simulink model "nonlinear_pid"  (R2021b)
settings: Solver=VariableStepAuto  StartTime=0.0  StopTime=60  RelTol=1e-3
libraries: slpidlib x6
settings Model: Creator=QP  LastModifiedBy=QP

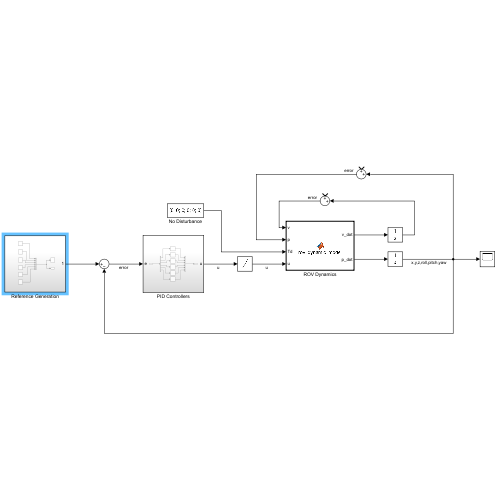
[thumbnail: Simulink's stored preview of the top-level diagram]
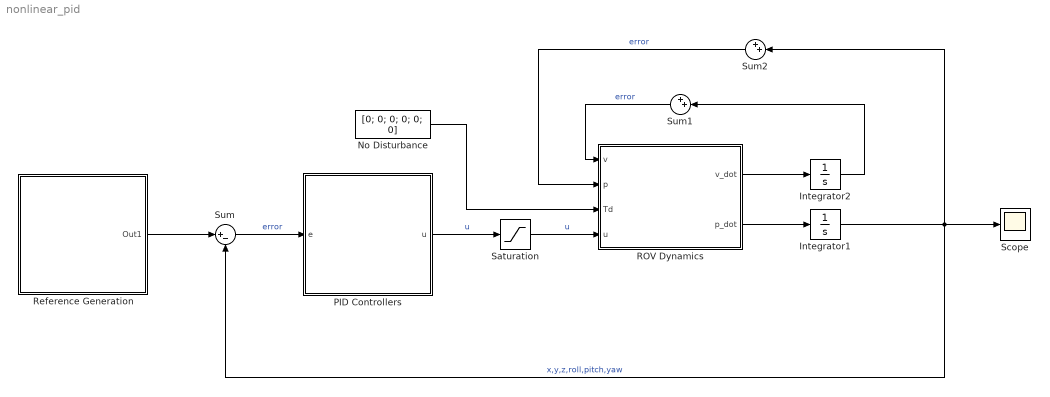
== system nonlinear_pid ==
  Integrator1 : Integrator
  Integrator2 : Integrator
  No Disturbance : Constant  Value=[0; 0; 0; 0; 0; 0]
  PID Controllers : Subsystem
  ROV Dynamics : MATLAB Function  TreatAsAtomicUnit=on
  Reference Generation : Subsystem
  Saturation : Saturate  UpperLimit=1  LowerLimit=-1
  Scope : Scope
  Sum : Sum  Inputs=|+-
  Sum1 : Sum  Inputs=++|
  Sum2 : Sum  Inputs=++|
  wires:
  PID Controllers/1(u) -> Saturation/1  "u"
  Reference Generation/1(Out1) -> Sum/1
  Sum/1 -> PID Controllers/1(e)  "error"
  Saturation/1 -> ROV Dynamics/4(u)  "u"
  No Disturbance/1 -> ROV Dynamics/3(Td)
  ROV Dynamics/2(p_dot) -> Integrator1/1
  ROV Dynamics/1(v_dot) -> Integrator2/1
  Integrator1/1 -> Sum2/2, Scope/1, Sum/2  "x,y,z,roll,pitch,yaw"
  Integrator2/1 -> Sum1/2
  Sum1/1 -> ROV Dynamics/1(v)  "error"
  Sum2/1 -> ROV Dynamics/2(p)  "error"

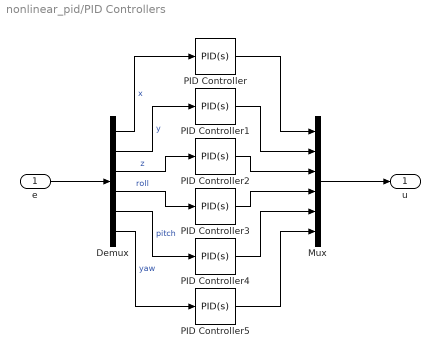
== system nonlinear_pid/PID Controllers ==
  e : Inport
  Demux : Demux  Outputs=6
  Mux : Mux  Inputs=6
  PID Controller{,3..5} (4 alike) : slpidlib/PID Controller  Controller=PID  Form=Parallel  TimeDomain=Continuous-time  UseExternalTs=off  SampleTime=-1  IntegratorMethod=Forward Euler  FilterMethod=Forward Euler  ControllerParametersSource=internal  P=1  I=0  D=0  UseFilter=on  N=100  TunerSelectOption=Transfer Function Based (PID Tuner App)  InitialConditionSource=internal  InitialConditionForIntegrator=0  InitialConditionForFilter=0  DifferentiatorICPrevScaledInput=0  ExternalReset=none  TrackingMode=off  Kt=1  LimitOutput=off  SatLimitsSource=internal  UpperSaturationLimit=inf  LowerSaturationLimit=-inf  LinearizeAsGain=on  AntiWindupMode=none  Kb=1  POutMin=[]  POutMax=[]  IOutMin=[]  IOutMax=[]  DOutMin=[]  DOutMax=[]  NOutMin=[]  NOutMax=[]  SumOutMin=[]  SumOutMax=[]  SaturationOutMin=[]  SaturationOutMax=[]  PParamMin=[]  PParamMax=[]  IParamMin=[]  IParamMax=[]  DParamMin=[]  DParamMax=[]  NParamMin=[]  NParamMax=[]  KbParamMin=[]  KbParamMax=[]  KtParamMin=[]  KtParamMax=[]  KbOutMin=[]  KbOutMax=[]  KtOutMin=[]  KtOutMax=[]  IntegratorOutMin=[]  IntegratorOutMax=[]  FilterOutMin=[]  FilterOutMax=[]  SumI1OutMin=[]  SumI1OutMax=[]  SumI2OutMin=[]  SumI2OutMax=[]  SumI3OutMin=[]  SumI3OutMax=[]  SumI4OutMin=[]  SumI4OutMax=[]  SumDOutMin=[]  SumDOutMax=[]  DifferentiatorOutMin=[]  DifferentiatorOutMax=[]  FilterDiffOutCoefMin=[]  FilterDiffOutCoefMax=[]  ReciprocalOutMin=[]  ReciprocalOutMax=[]  SumDenOutMin=[]  SumDenOutMax=[]  SumNumOutMin=[]  SumNumOutMax=[]  DivideOutMin=[]  DivideOutMax=[]  UdiffTsProdOutMin=[]  UdiffTsProdOutMax=[]  NTsProdOutMin=[]  NTsProdOutMax=[]  UintegralTsProdOutMin=[]  UintegralTsProdOutMax=[]  UngainTsProdOutMin=[]  UngainTsProdOutMax=[]  IntegratorContinuousStateAttributes=''  IntegratorStateMustResolveToSignalObject=off  IntegratorRTWStateStorageClass=Auto  FilterContinuousStateAttributes=''  FilterStateMustResolveToSignalObject=off  FilterRTWStateStorageClass=Auto  ParallelPVariant=InternalParameters  IdealPVariant=Disabled  IVariant=InternalParameters  DVariant=InternalParameters  IntegratorVariant=Continuous  SatVariant=Disabled  AWVariant=Passthrough  PCopyVariant=Disabled  TRVariant=Disabled  FdbkBlocksVariant=Forward  IdealPFdbkVariant=Disabled  SatFdbkVariant=Disabled  DerivativeFilterVariant=ContFilter  NVariant=InternalParameters  NCopyVariant=Disabled  FilterICVariant=InternalICsFilter  IntegratorICVariant=InternalICs  ExternalResetVariant=Disabled  TRSumVariant=Passthrough  SumFdbkVariant=Disabled  SumVariant=Sum_PID  TsampFilterVariant=InternalTs  TsampNgainVariant=Passthrough  TsampIntegralVariant=Passthrough  ExternalSaturationOutDataTypeStr=Inherit: Same as second input
  PID Controller1 : slpidlib/PID Controller  Controller=PID  Form=Parallel  TimeDomain=Continuous-time  UseExternalTs=off  SampleTime=-1  IntegratorMethod=Forward Euler  FilterMethod=Forward Euler  ControllerParametersSource=internal  P=1  I=1  D=0  UseFilter=on  N=100  TunerSelectOption=Transfer Function Based (PID Tuner App)  InitialConditionSource=internal  InitialConditionForIntegrator=0  InitialConditionForFilter=0  DifferentiatorICPrevScaledInput=0  ExternalReset=none  TrackingMode=off  Kt=1  LimitOutput=off  SatLimitsSource=internal  UpperSaturationLimit=inf  LowerSaturationLimit=-inf  LinearizeAsGain=on  AntiWindupMode=none  Kb=1  POutMin=[]  POutMax=[]  IOutMin=[]  IOutMax=[]  DOutMin=[]  DOutMax=[]  NOutMin=[]  NOutMax=[]  SumOutMin=[]  SumOutMax=[]  SaturationOutMin=[]  SaturationOutMax=[]  PParamMin=[]  PParamMax=[]  IParamMin=[]  IParamMax=[]  DParamMin=[]  DParamMax=[]  NParamMin=[]  NParamMax=[]  KbParamMin=[]  KbParamMax=[]  KtParamMin=[]  KtParamMax=[]  KbOutMin=[]  KbOutMax=[]  KtOutMin=[]  KtOutMax=[]  IntegratorOutMin=[]  IntegratorOutMax=[]  FilterOutMin=[]  FilterOutMax=[]  SumI1OutMin=[]  SumI1OutMax=[]  SumI2OutMin=[]  SumI2OutMax=[]  SumI3OutMin=[]  SumI3OutMax=[]  SumI4OutMin=[]  SumI4OutMax=[]  SumDOutMin=[]  SumDOutMax=[]  DifferentiatorOutMin=[]  DifferentiatorOutMax=[]  FilterDiffOutCoefMin=[]  FilterDiffOutCoefMax=[]  ReciprocalOutMin=[]  ReciprocalOutMax=[]  SumDenOutMin=[]  SumDenOutMax=[]  SumNumOutMin=[]  SumNumOutMax=[]  DivideOutMin=[]  DivideOutMax=[]  UdiffTsProdOutMin=[]  UdiffTsProdOutMax=[]  NTsProdOutMin=[]  NTsProdOutMax=[]  UintegralTsProdOutMin=[]  UintegralTsProdOutMax=[]  UngainTsProdOutMin=[]  UngainTsProdOutMax=[]  IntegratorContinuousStateAttributes=''  IntegratorStateMustResolveToSignalObject=off  IntegratorRTWStateStorageClass=Auto  FilterContinuousStateAttributes=''  FilterStateMustResolveToSignalObject=off  FilterRTWStateStorageClass=Auto  ParallelPVariant=InternalParameters  IdealPVariant=Disabled  IVariant=InternalParameters  DVariant=InternalParameters  IntegratorVariant=Continuous  SatVariant=Disabled  AWVariant=Passthrough  PCopyVariant=Disabled  TRVariant=Disabled  FdbkBlocksVariant=Forward  IdealPFdbkVariant=Disabled  SatFdbkVariant=Disabled  DerivativeFilterVariant=ContFilter  NVariant=InternalParameters  NCopyVariant=Disabled  FilterICVariant=InternalICsFilter  IntegratorICVariant=InternalICs  ExternalResetVariant=Disabled  TRSumVariant=Passthrough  SumFdbkVariant=Disabled  SumVariant=Sum_PID  TsampFilterVariant=InternalTs  TsampNgainVariant=Passthrough  TsampIntegralVariant=Passthrough  ExternalSaturationOutDataTypeStr=Inherit: Same as second input
  PID Controller2 : slpidlib/PID Controller  Controller=PID  Form=Parallel  TimeDomain=Continuous-time  UseExternalTs=off  SampleTime=-1  IntegratorMethod=Forward Euler  FilterMethod=Forward Euler  ControllerParametersSource=internal  P=1.5  I=0.02  D=0  UseFilter=on  N=12.9464363857845  TunerSelectOption=Transfer Function Based (PID Tuner App)  InitialConditionSource=internal  InitialConditionForIntegrator=0  InitialConditionForFilter=0  DifferentiatorICPrevScaledInput=0  ExternalReset=none  TrackingMode=off  Kt=1  LimitOutput=off  SatLimitsSource=internal  UpperSaturationLimit=inf  LowerSaturationLimit=-inf  LinearizeAsGain=on  AntiWindupMode=none  Kb=1  POutMin=[]  POutMax=[]  IOutMin=[]  IOutMax=[]  DOutMin=[]  DOutMax=[]  NOutMin=[]  NOutMax=[]  SumOutMin=[]  SumOutMax=[]  SaturationOutMin=[]  SaturationOutMax=[]  PParamMin=[]  PParamMax=[]  IParamMin=[]  IParamMax=[]  DParamMin=[]  DParamMax=[]  NParamMin=[]  NParamMax=[]  KbParamMin=[]  KbParamMax=[]  KtParamMin=[]  KtParamMax=[]  KbOutMin=[]  KbOutMax=[]  KtOutMin=[]  KtOutMax=[]  IntegratorOutMin=[]  IntegratorOutMax=[]  FilterOutMin=[]  FilterOutMax=[]  SumI1OutMin=[]  SumI1OutMax=[]  SumI2OutMin=[]  SumI2OutMax=[]  SumI3OutMin=[]  SumI3OutMax=[]  SumI4OutMin=[]  SumI4OutMax=[]  SumDOutMin=[]  SumDOutMax=[]  DifferentiatorOutMin=[]  DifferentiatorOutMax=[]  FilterDiffOutCoefMin=[]  FilterDiffOutCoefMax=[]  ReciprocalOutMin=[]  ReciprocalOutMax=[]  SumDenOutMin=[]  SumDenOutMax=[]  SumNumOutMin=[]  SumNumOutMax=[]  DivideOutMin=[]  DivideOutMax=[]  UdiffTsProdOutMin=[]  UdiffTsProdOutMax=[]  NTsProdOutMin=[]  NTsProdOutMax=[]  UintegralTsProdOutMin=[]  UintegralTsProdOutMax=[]  UngainTsProdOutMin=[]  UngainTsProdOutMax=[]  IntegratorContinuousStateAttributes=''  IntegratorStateMustResolveToSignalObject=off  IntegratorRTWStateStorageClass=Auto  FilterContinuousStateAttributes=''  FilterStateMustResolveToSignalObject=off  FilterRTWStateStorageClass=Auto  ParallelPVariant=InternalParameters  IdealPVariant=Disabled  IVariant=InternalParameters  DVariant=InternalParameters  IntegratorVariant=Continuous  SatVariant=Disabled  AWVariant=Passthrough  PCopyVariant=Disabled  TRVariant=Disabled  FdbkBlocksVariant=Forward  IdealPFdbkVariant=Disabled  SatFdbkVariant=Disabled  DerivativeFilterVariant=ContFilter  NVariant=InternalParameters  NCopyVariant=Disabled  FilterICVariant=InternalICsFilter  IntegratorICVariant=InternalICs  ExternalResetVariant=Disabled  TRSumVariant=Passthrough  SumFdbkVariant=Disabled  SumVariant=Sum_PID  TsampFilterVariant=InternalTs  TsampNgainVariant=Passthrough  TsampIntegralVariant=Passthrough  ExternalSaturationOutDataTypeStr=Inherit: Same as second input
  u : Outport
  wires:
  e/1 -> Demux/1
  Mux/1 -> u/1
  PID Controller/1 -> Mux/1
  Demux/1 -> PID Controller/1  "x"
  Demux/6 -> PID Controller5/1  "yaw"
  PID Controller5/1 -> Mux/6
  PID Controller4/1 -> Mux/5
  Demux/5 -> PID Controller4/1  "pitch"
  Demux/2 -> PID Controller1/1  "y"
  PID Controller1/1 -> Mux/2
  Demux/3 -> PID Controller2/1  "z"
  Demux/4 -> PID Controller3/1  "roll"
  PID Controller2/1 -> Mux/3
  PID Controller3/1 -> Mux/4

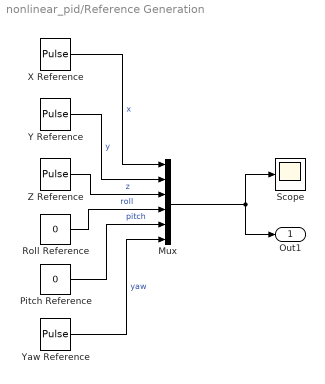
== system nonlinear_pid/Reference Generation ==
  Mux : Mux  Inputs=6
  Pitch Reference : Constant  Value=0
  Roll Reference : Constant  Value=0
  Scope : Scope
  X Reference : DiscretePulseGenerator  PulseType=Time based  Amplitude=0  Period=70  PulseWidth=20/70*100  PhaseDelay=15
  Y Reference : DiscretePulseGenerator  PulseType=Time based  Amplitude=0  Period=70  PulseWidth=20/70*100  PhaseDelay=25
  Yaw Reference : DiscretePulseGenerator  PulseType=Time based  Amplitude=0  Period=70  PulseWidth=10/70*100
  Z Reference : DiscretePulseGenerator  PulseType=Time based  Amplitude=-3  Period=300  PulseWidth=99  PhaseDelay=5
  Out1 : Outport
  wires:
  Mux/1 -> Scope/1, Out1/1
  X Reference/1 -> Mux/1  "x"
  Yaw Reference/1 -> Mux/6  "yaw"
  Y Reference/1 -> Mux/2  "y"
  Pitch Reference/1 -> Mux/5  "pitch"
  Z Reference/1 -> Mux/3  "z"
  Roll Reference/1 -> Mux/4  "roll"

== matlab function nonlinear_pid/ROV Dynamics ==
  data: v input; p input; v_dot output; p_dot output; Td input; u input
function [v_dot, p_dot] = rov_dynamic_model(v, p, Td, u)

v_dot = zeros([6, 1]);
p_dot = zeros([6, 1]);

% BlueROV2 Heavy Configuration Specifications 

g = 9.82;    % m/s^2
rho = 1000;  % kg/m3

m = 13.5;    % kg
V = 0.0134;  % m^3

Ix = 0.26;  % kg*m2
Iy = 0.23;  % kg*m2
Iz = 0.37;  % kg*m2

g_center =  [0, 0, 0];      % m
b_center =  [0, 0, -0.01];  % m

Xu_l = 13.7;   % Ns/m (Linear drag surge)
Yv_l = 0;      % Ns/m (Linear drag sway)
Zw_l = 33.0;   % Ns/m (Linear drag heave)
Kp_l = 0;      % Ns/m (Linear drag roll)
Mq_l = 0.8;    % Ns/m (Linear drag pitch)
Nr_l = 0;      % Ns/m (Linear drag yaw)

Xu_q = 141.0;  % Ns^2/m^2 (Quadratic drag surge)
Yv_q = 217.0;  % Ns^2/m^2 (Quadratic drag sway)
Zw_q = 190.0;  % Ns^2/m^2 (Quadratic drag heave)
Kp_q = 1.19;   % Ns^2/m^2 (Quadratic drag roll)
Mq_q = 0.47;   % Ns^2/m^2 (Quadratic drag pitch)
Nr_q = 1.5;    % Ns^2/m^2 (Quadratic drag yaw)

Xu_a = 6.36;   % kg (Added mass surge)
Yv_a = 7.12;   % kg (Added mass sway)
Zw_a = 18.68;  % kg (Added mass heave)
Kp_a = 0.189;  % kg*m^2 (Added mass roll)
Mq_a = 0.135;  % kg*m^2 (Added mass pitch)
Nr_a = 0.222;  % kg*m^2 (Added mass yaw)


% ------------------------------Dynamics-----------------------------------


M_rb = eye(6).*[m, m, m, Ix, Iy, Iz];                % Rigid body mass
M_a = eye(6).*[Xu_a, Yv_a, Zw_a, Kp_a, Mq_a, Nr_a];  % Added mass
M = M_rb + M_a;  % Mass Matrix

D_l = eye(6).*[Xu_l, Yv_l, Zw_l, Kp_l, Mq_l, Nr_l];  % Linear drag matrix
D_q = eye(6).*[Xu_q, Yv_q, Zw_q, Kp_q, Mq_q, Nr_q];  % Quadratic drag matrix
D = D_l + D_q;  % Hydrodynamic damping

W = m*g;      % Weight
B = rho*g*V;  % Buoyancy

x_g = g_center(1);
y_g = g_center(2);
z_g = g_center(3);
x_b = b_center(1);
y_b = b_center(2);
z_b = b_center(3);

% Restoring force
g_n = [                    (W-B)*sin(p(5,1));
                     -(W-B)*cos(p(5,1))*sin(p(4,1));
                     -(W-B)*cos(p(5,1))*cos(p(4,1));
  -(y_g*W-y_b*B)*cos(p(5,1))*cos(p(4,1)) + (z_g*W-z_b*B)*cos(p(5,1))*sin(p(4,1));
        (z_g*W-z_b*B)*sin(p(5,1)) + (x_g*W-x_b*B)*cos(p(5,1))*cos(p(4,1));
       -(x_g*W-x_b*B)*cos(p(5,1))*sin(p(4,1)) - (y_g*W-y_b*B)*sin(p(5,1)) ];

% Thruster allocation matrix
K = [ 0.7071,  0.7071, -0.7071, -0.7071,       0,       0,       0,       0;
     -0.7071,  0.7071, -0.7071,  0.7071,       0,       0,       0,       0;
           0,       0,       0,       0, -1.0000, -1.0000, -1.0000, -1.0000;
           0,       0,       0,       0,  0.2180,  0.2180, -0.2180, -0.2180;
           0,       0,       0,       0,  0.1200, -0.1200,  0.1200, -0.1200;
     -0.1888,  0.1888,  0.1888, -0.1888,       0,       0,       0,       0 ];

% Control allocation matrix
A = [-1,  1,  0,  0,  0,  1;
     -1, -1,  0,  0,  0, -1;
      1,  1,  0,  0,  0, -1;
      1, -1,  0,  0,  0,  1;
      0,  0, -1, -1,  1,  0;
      0,  0, -1,  1,  1,  0;
      0,  0, -1,  1, -1,  0;
      0,  0, -1, -1, -1,  0 ];

a = A*u;                              % Allocated control signal
t = (80 ./ ( 1 + exp(-4.*a.^3) )) - 40;  % Thrust
To = K*t;  % Force and moment from propellers

v_dot = M^(-1) * (To + Td - D*v - g_n);


% -----------------------------Kinematics----------------------------------


% Transformation matrix of linear velocity
R_n = zeros([3, 3]);

R_n(1, 1) = cos(p(4,1))*cos(p(5,1));
R_n(1, 2) = -sin(p(6,1))*cos(p(4,1)) + cos(p(6,1))*sin(p(5,1))*sin(p(4,1));
R_n(1, 3) = sin(p(6,1))*sin(p(4,1)) + cos(p(6,1))*cos(p(4,1))*sin(p(5,1));

R_n(2, 1) = sin(p(4,1))*cos(p(5,1));
R_n(2, 2) = cos(p(6,1))*cos(p(4,1)) + sin(p(4,1))*sin(p(5,1))*sin(p(6,1));
R_n(2, 3) = -cos(p(6,1))*sin(p(4,1)) + sin(p(5,1))*sin(p(6,1))*cos(p(4,1));

R_n(3, 1) = -sin(p(5,1));
R_n(3, 2) = cos(p(5,1))*sin(p(4,1));
R_n(3, 3) = cos(p(5,1))*cos(p(4,1));

% Transformation matrix of angular velocity
T_n = zeros([3, 3]);

T_n(1, 1) = 1;
T_n(1, 2) = sin(p(6,1))*sin(p(5,1))/cos(p(5,1));
T_n(1, 3) = cos(p(4,1))*sin(p(5,1))/cos(p(5,1));

T_n(2, 1) = 0;
T_n(2, 2) = cos(p(4,1));
T_n(2, 3) = sin(p(4,1));

T_n(3, 1) = 0;
T_n(3, 2) = sin(p(4,1))/cos(p(5,1));
T_n(3, 3) = cos(p(4,1))/cos(p(5,1));

J_n = [R_n, zeros([3,3]); zeros([3,3]), T_n];  % Transformation to the body velocity

p_dot = J_n * v;
